simulink library "motdrv_lib"  (Simulink 7.6)
settings: Solver=ode45  StartTime=0.0  StopTime=10.0  RelTol=1e-3
settings Model: Creator=dauger  LastModifiedBy=dauger

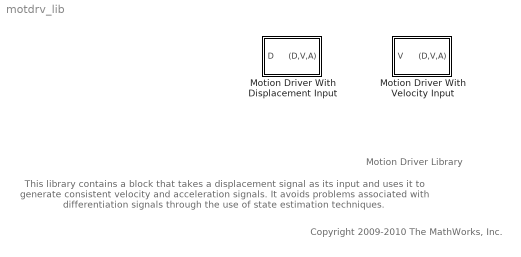
== system motdrv_lib ==
  note: Motion Driver Library
  note: This library contains a block that takes a displacement signal as its input and
      | uses it to generate consistent velocity and acceleration signals.  It avoids problems
      | associated with differentiation signals through the use of state estimation techniques.
  note: Copyright 2009-2010 The MathWorks, Inc.
  Motion Driver With Displacement Input : Subsystem  mask(Motion Driver with Acceleration Input){InitialDisplacementSource=Dialog, InitialDisplacement=0, InitialVelocity=0, TimeConstant=1}
      mask prompts: InitialDisplacementSource "Initial displacement source:"; InitialDisplacement "Initial Displacement (units):"; InitialVelocity "Initial Velocity (units/s):"; TimeConstant "Time Constant (s):"
      mask help: This block takes as its input an acceleration and produces a three-dimensional output vector containing a displacement, a velocity and the original acceleration. This is useful for driving SimMechanics actuators with motion. To get correct performance, the user needs to specify the initial displacement and velocity signals. (The displacement can be inherited from the initial input.)
      mask init:
      | if InitialDisplacementSource == 2 % INHERITED
      |     InitialDisplacement = 0;
      | end
      mask StyleString: popup(Dialog|Inherited),edit,edit,edit
      mask CallbackString: motdrv_lib_callbacks(gcb(), 'INITIAL_DISPLACEMENT_SOURCE_DIALOG_CALLBACK');|||
      mask Display:
      | port_label('input', 1, 'D');
      | port_label('output', 1, '(D,V,A)');
  Motion Driver With Velocity Input : Subsystem  mask(Motion Driver with Acceleration Input){InitialDisplacement=0, InitialVelocitySource=Dialog, InitialVelocity=0, TimeConstant=1}
      mask prompts: InitialDisplacement "Initial Displacement (units):"; InitialVelocitySource "Initial velocity source:"; InitialVelocity "Initial Velocity (units/s):"; TimeConstant "Time Constant (s):"
      mask help: This block takes as its input an acceleration and produces a three-dimensional output vector containing a displacement, a velocity and the original acceleration. This is useful for driving SimMechanics actuators with motion. To get correct performance, the user needs to specify the initial displacement and velocity signals. (The displacement can be inherited from the initial input.)
      mask init:
      | if InitialVelocitySource == 2 % INHERITED
      |     InitialVelocity = 0;
      | end
      mask StyleString: edit,popup(Dialog|Inherited),edit,edit
      mask CallbackString: |motdrv_lib_callbacks(gcb(), 'INITIAL_VELOCITY_SOURCE_DIALOG_CALLBACK');||
      mask Display:
      | port_label('input', 1, 'V');
      | port_label('output', 1, '(D,V,A)');

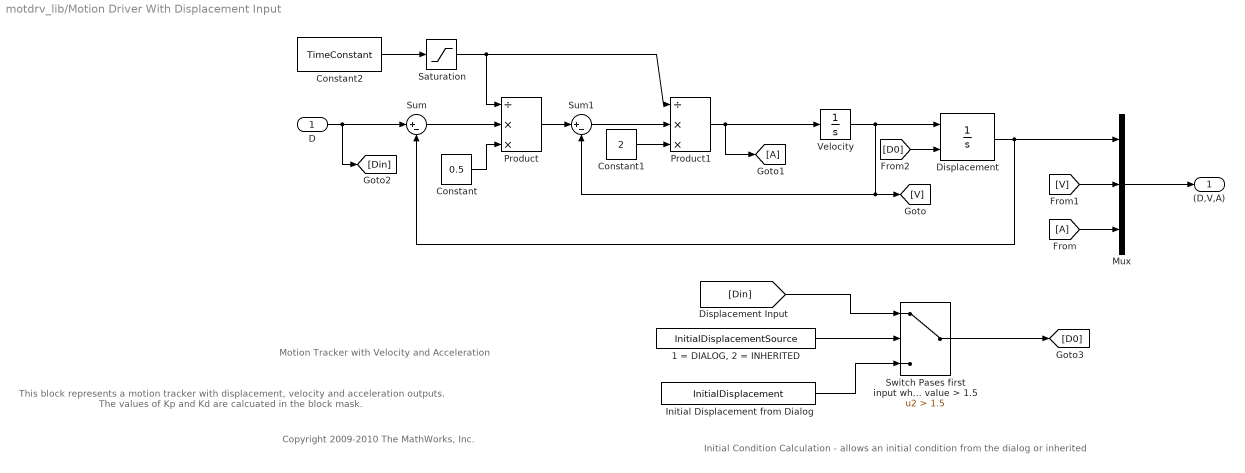
== system motdrv_lib/Motion Driver With Displacement Input ==
  note: Initial Condition Calculation - allows an initial condition from the dialog or inherited
  note: Motion Tracker with Velocity and Acceleration
  note: This block represents a motion tracker with displacement, velocity
      | and acceleration outputs.  The values of Kp and Kd are calcuated
      | in the block mask.
  note: Copyright 2009-2010 The MathWorks, Inc.
  D : Inport  PortDimensions=1
  "1 = DIALOG, 2 = INHERITED" : Constant  Value=InitialDisplacementSource
  Constant : Constant  Value=0.5
  Constant1 : Constant  Value=2
  Constant2 : Constant  Value=TimeConstant
  Displacement : Integrator  InitialConditionSource=external
  Initial Displacement from Dialog : Constant  Value=InitialDisplacement
  Mux : Mux  Inputs=3
  Product : Product  Inputs=/**  RndMeth=Zero
  Product1 : Product  Inputs=/**  RndMeth=Zero
  Saturation : Saturate  UpperLimit=Inf  LowerLimit=eps
      settings: AttributesFormatString=Upper Limit = %<UpperLimit>\nLower Limit = %<LowerLimit>
  Sum : Sum  Inputs=|+-
  Sum1 : Sum  Inputs=|+-
  Switch Pases first input when switching value > 1.5 : Switch  Criteria=u2 > Threshold  Threshold=1.5
  Velocity : Integrator  InitialCondition=InitialVelocity
  (D,V,A) : Outport  PortDimensions=3
  wires:
  [D0] -> Displacement/2
  Switch Pases first input when switching value > 1.5/1 -> [D0]
  Initial Displacement from Dialog/1 -> Switch Pases first input when switching value > 1.5/3
  [Din] -> Switch Pases first input when switching value > 1.5/1
  "1 = DIALOG, 2 = INHERITED"/1 -> Switch Pases first input when switching value > 1.5/2
  D/1 -> [Din], Sum/1
  Sum/1 -> Product/2
  Sum1/1 -> Product1/2
  Mux/1 -> (D,V,A)/1
  Displacement/1 -> Mux/1, Sum/2
  Velocity/1 -> Displacement/1, Sum1/2, [V]
  Product/1 -> Sum1/1
  Product1/1 -> [A], Velocity/1
  Constant/1 -> Product/3
  Constant1/1 -> Product1/3
  Constant2/1 -> Saturation/1
  Saturation/1 -> Product/1, Product1/1
  [V] -> Mux/2
  [A] -> Mux/3

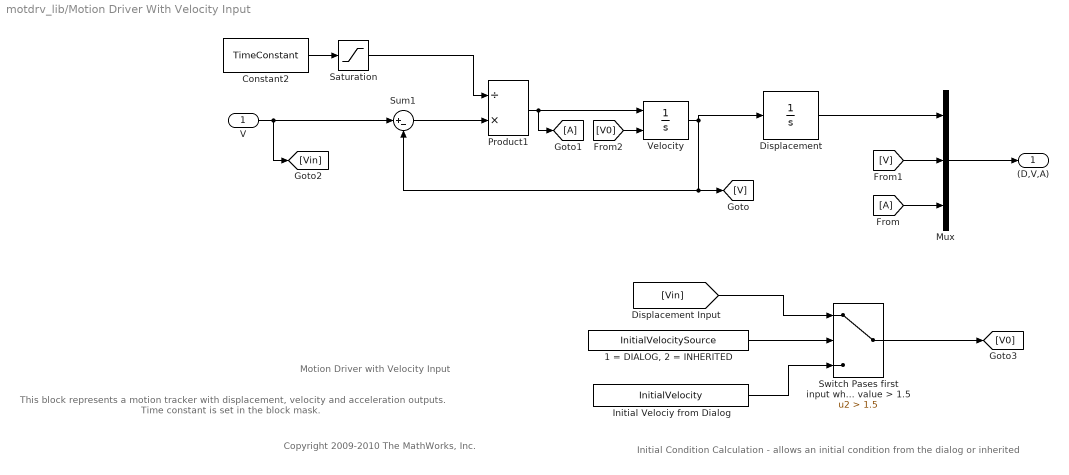
== system motdrv_lib/Motion Driver With Velocity Input ==
  note: Copyright 2009-2010 The MathWorks, Inc.
  note: This block represents a motion tracker with displacement, velocity
      | and acceleration outputs.  Time constant is set in the block mask.
  note: Motion Driver with Velocity Input
  note: Initial Condition Calculation - allows an initial condition from the dialog or inherited
  V : Inport  PortDimensions=1
  "1 = DIALOG, 2 = INHERITED" : Constant  Value=InitialVelocitySource
  Constant2 : Constant  Value=TimeConstant
  Displacement : Integrator  InitialCondition=InitialDisplacement
  Initial Velociy from Dialog : Constant  Value=InitialVelocity
  Mux : Mux  Inputs=3
  Product1 : Product  Inputs=/*  RndMeth=Zero
  Saturation : Saturate  UpperLimit=Inf  LowerLimit=eps
      settings: AttributesFormatString=Upper Limit = %<UpperLimit>\nLower Limit = %<LowerLimit>
  Sum1 : Sum  Inputs=|+-
  Switch Pases first input when switching value > 1.5 : Switch  Criteria=u2 > Threshold  Threshold=1.5
  Velocity : Integrator  InitialConditionSource=external
  (D,V,A) : Outport  PortDimensions=3
  wires:
  [A] -> Mux/3
  [V] -> Mux/2
  Saturation/1 -> Product1/1
  Constant2/1 -> Saturation/1
  Product1/1 -> Velocity/1, [A]
  Velocity/1 -> [V], Sum1/2, Displacement/1
  Displacement/1 -> Mux/1
  Mux/1 -> (D,V,A)/1
  Sum1/1 -> Product1/2
  V/1 -> [Vin], Sum1/1
  "1 = DIALOG, 2 = INHERITED"/1 -> Switch Pases first input when switching value > 1.5/2
  [Vin] -> Switch Pases first input when switching value > 1.5/1
  Initial Velociy from Dialog/1 -> Switch Pases first input when switching value > 1.5/3
  Switch Pases first input when switching value > 1.5/1 -> [V0]
  [V0] -> Velocity/2
